simulink model "single_track"  (R2021a)
settings: Solver=VariableStepAuto  StartTime=0.0  StopTime=80  FixedStep=0.001  RelTol=1e-3
libraries: pid_lib x1
settings Model: Creator=ouafo  LastModifiedBy=ouafo

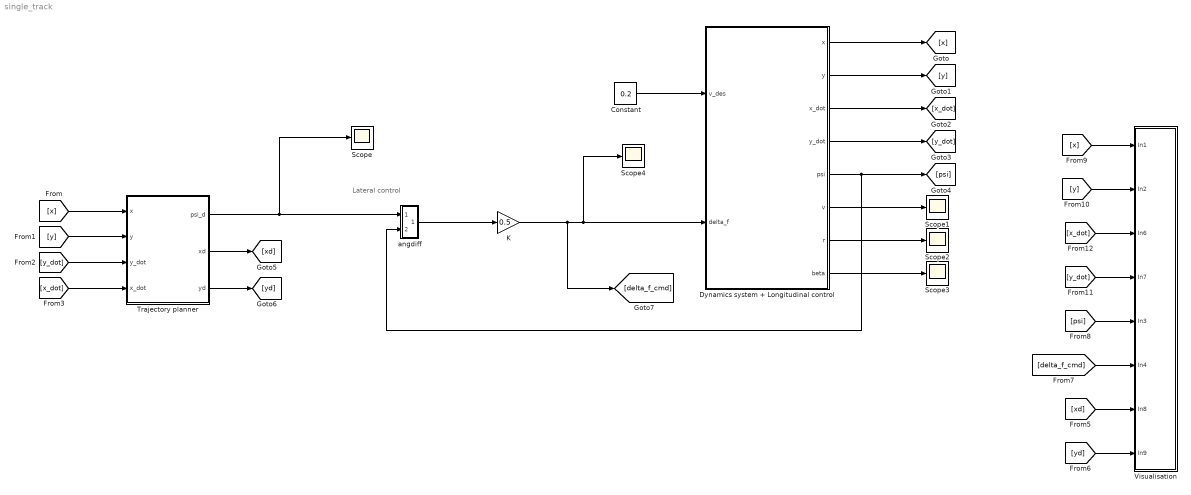
== system single_track ==
  note: Lateral control
  Constant : Constant  Value=0.2
  Dynamics system + Longitudinal control : Subsystem
  K : Gain  Gain=0.5
  Scope{,1..4} (5 alike) : Scope
  Trajectory planner : Subsystem
  Visualisation : Subsystem
  angdiff : Subsystem
  wires:
  Constant/1 -> Dynamics system + Longitudinal control/1(v_des)
  Dynamics system + Longitudinal control/1(x) -> [x]
  Dynamics system + Longitudinal control/2(y) -> [y]
  Dynamics system + Longitudinal control/3(x_dot) -> [x_dot]
  Dynamics system + Longitudinal control/4(y_dot) -> [y_dot]
  Dynamics system + Longitudinal control/5(psi) -> angdiff/2(-), [psi]
  Dynamics system + Longitudinal control/6(v) -> Scope1/1
  Dynamics system + Longitudinal control/7(r) -> Scope2/1
  Dynamics system + Longitudinal control/8(beta) -> Scope3/1
  [x] -> Trajectory planner/1(x)
  [y] -> Trajectory planner/2(y)
  [y_dot] -> Trajectory planner/3(y_dot)
  [x_dot] -> Trajectory planner/4(x_dot)
  Trajectory planner/2(xd) -> [xd]
  Trajectory planner/3(yd) -> [yd]
  angdiff/1(e) -> K/1
  [x] -> Visualisation/1(In1)
  [y] -> Visualisation/2(In2)
  [yd] -> Visualisation/8(In9)
  [xd] -> Visualisation/7(In8)
  [x_dot] -> Visualisation/3(In6)
  [y_dot] -> Visualisation/4(In7)
  [delta_f_cmd] -> Visualisation/6(In4)
  [psi] -> Visualisation/5(In3)
  Trajectory planner/1(psi_d) -> Scope/1, angdiff/1(+)
  K/1 -> [delta_f_cmd], Scope4/1, Dynamics system + Longitudinal control/2(delta_f)

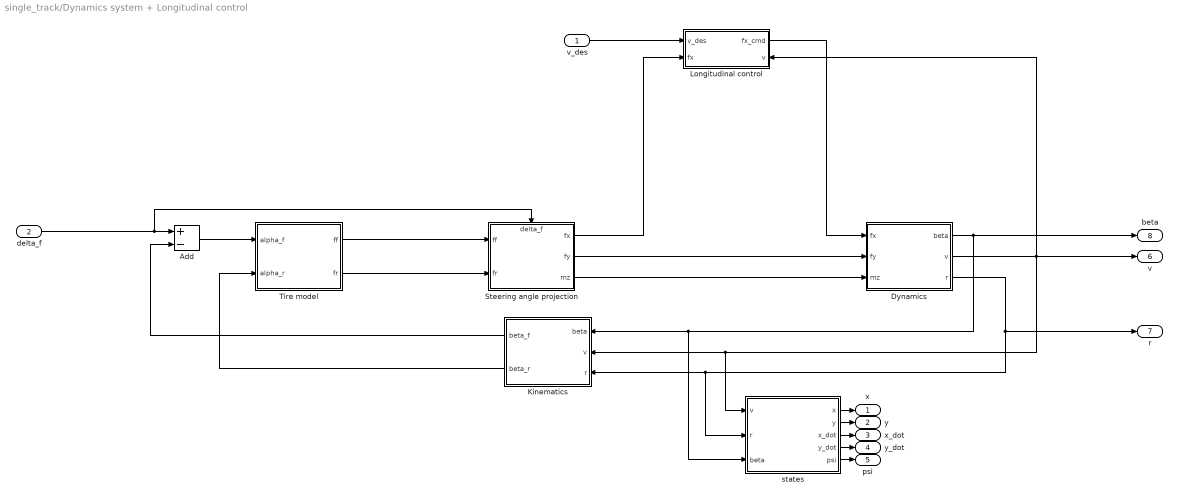
== system single_track/Dynamics system + Longitudinal control ==
  v_des : Inport
  delta_f : Inport  Port=2
  Add : Sum  Inputs=+-
  Dynamics : Subsystem
  Kinematics : Subsystem
  Longitudinal control : Subsystem
      settings: PortSchema="{\"entries\":[{\"content\":{\"sides\":[{\"content\":{\"connectorIds\":[\"In1\",\"In2\"]},\"type\":\"ConnectorPlacement.EquallySpacedRectSide\",\"uuid\":\"998833cc-1ae3-458a-8afb-96cc18db8c80\"},{\"content\":{\"connectorIds\":[\"Out1\",\"In3\"],\"side\":\"RIGHT\"},\"type\":\"ConnectorPlacement.EquallySpacedRectSide\",\"uuid\":\"fcb5fd6e-7c15-4d63-8239-7525f445e8c5\"},{\"content\":{\"connectorIds\":[],\"side\":\"TOP\"},\"type\":\"ConnectorPlacement.EquallySpacedRectSide\",\"uuid\":\"70c6e347-3bc2-4202-b834-379cf179dd08\"},{\"content\":{\"connectorIds\":[],\"side\":\"BOTTOM\"},\"type\":\"ConnectorPlacement.EquallySpacedRectSide\",\"uuid\":\"2cc4168b-3eb3-494f-b0d0-8a728c963cb1\"}]},\"type\":\"ConnectorPlacement.EquallySpacedConnector\",\"uuid\":\"1cd2931d-9394-40f3-bda0-3ecfedd53b05\"}],\"packageUris\":[\"http://schema.mathworks.com/mf0/Connector/R2020b\"],\"version\":\"1.0\"}"
  Steering angle projection : Subsystem
      settings: PortSchema="{\"entries\":[{\"content\":{\"sides\":[{\"content\":{\"connectorIds\":[\"In1\",\"In2\"]},\"type\":\"ConnectorPlacement.EquallySpacedRectSide\",\"uuid\":\"851b8f0b-7850-4432-b3a6-e49d1b849a22\"},{\"content\":{\"connectorIds\":[\"Out1\",\"Out2\",\"Out3\"],\"side\":\"RIGHT\"},\"type\":\"ConnectorPlacement.EquallySpacedRectSide\",\"uuid\":\"60b21c17-1cf9-454c-9b20-5b400b47ede1\"},{\"content\":{\"connectorIds\":[\"In3\"],\"side\":\"TOP\"},\"type\":\"ConnectorPlacement.EquallySpacedRectSide\",\"uuid\":\"9c5c9653-2b7a-48f5-af80-1cee6375c418\"}]},\"type\":\"ConnectorPlacement.EquallySpacedConnector\",\"uuid\":\"bd97c71a-a528-4f5e-9945-06be100bb47e\"}],\"packageUris\":[\"http://schema.mathworks.com/mf0/Connector/R2020b\"],\"version\":\"1.0\"}"
  Tire model : Subsystem
  states : Subsystem
  x : Outport
  y : Outport  Port=2
  x_dot : Outport  Port=3
  y_dot : Outport  Port=4
  psi : Outport  Port=5
  v : Outport  Port=6
  r : Outport  Port=7
  beta : Outport  Port=8
  wires:
  Longitudinal control/1(fx_cmd) -> Dynamics/1(fx)
  Tire model/2(fr) -> Steering angle projection/2(fr)
  Tire model/1(ff) -> Steering angle projection/1(ff)
  states/1(x) -> x/1
  states/3(x_dot) -> x_dot/1
  delta_f/1 -> Steering angle projection/3(delta_f), Add/1
  Dynamics/2(v) -> v/1, states/1(v), Kinematics/2(v), Longitudinal control/3(v)
  Kinematics/1(beta_f) -> Add/2
  Kinematics/2(beta_r) -> Tire model/2(alpha_r)
  v_des/1 -> Longitudinal control/1(v_des)
  states/2(y) -> y/1
  Add/1 -> Tire model/1(alpha_f)
  Steering angle projection/3(mz) -> Dynamics/3(mz)
  states/4(y_dot) -> y_dot/1
  Dynamics/1(beta) -> beta/1, Kinematics/1(beta), states/3(beta)
  Steering angle projection/1(fx) -> Longitudinal control/2(fx)
  Dynamics/3(r) -> r/1, Kinematics/3(r), states/2(r)
  Steering angle projection/2(fy) -> Dynamics/2(fy)
  states/5(psi) -> psi/1

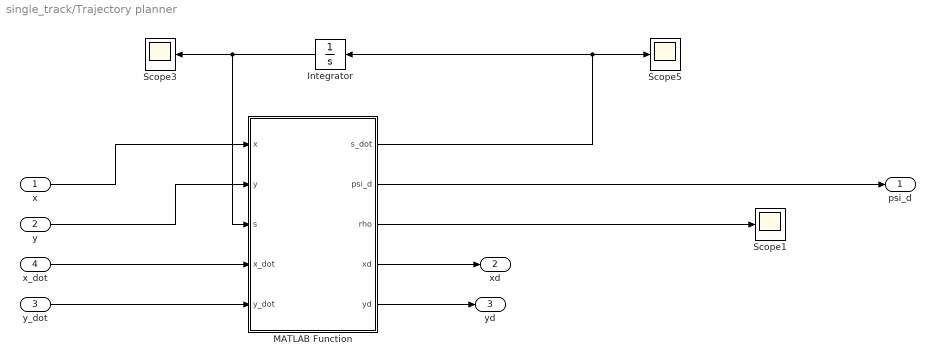
== system single_track/Trajectory planner ==
  x : Inport
  y : Inport  Port=2
  y_dot : Inport  Port=3
  x_dot : Inport  Port=4
  Integrator : Integrator  InitialCondition=-2
  MATLAB Function : MATLAB Function  TreatAsAtomicUnit=on
  Scope1 : Scope
  Scope3 : Scope
  Scope5 : Scope
  psi_d : Outport
  xd : Outport  Port=2
  yd : Outport  Port=3
  wires:
  x/1 -> MATLAB Function/1(x)
  y/1 -> MATLAB Function/2(y)
  y_dot/1 -> MATLAB Function/5(y_dot)
  x_dot/1 -> MATLAB Function/4(x_dot)
  MATLAB Function/1(s_dot) -> Integrator/1, Scope5/1
  Integrator/1 -> MATLAB Function/3(s), Scope3/1
  MATLAB Function/2(psi_d) -> psi_d/1
  MATLAB Function/3(rho) -> Scope1/1
  MATLAB Function/4(xd) -> xd/1
  MATLAB Function/5(yd) -> yd/1

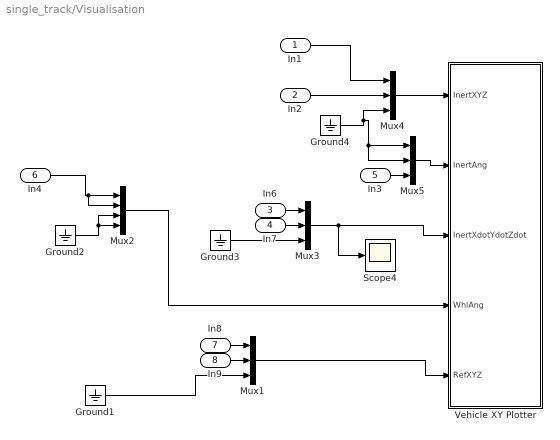
== system single_track/Visualisation ==
  In1 : Inport  PortDimensions=1
  In2 : Inport  Port=2  PortDimensions=1
  In6 : Inport  Port=3  PortDimensions=1
  In7 : Inport  Port=4  PortDimensions=1
  In3 : Inport  Port=5  PortDimensions=1
  In4 : Inport  Port=6  PortDimensions=1
  In8 : Inport  Port=7  PortDimensions=1
  In9 : Inport  Port=8  PortDimensions=1
  Ground{1..4} (4 alike) : Ground
  Mux{1,3..5} (4 alike) : Mux  Inputs=3
  Mux2 : Mux
  Scope4 : Scope
  Vehicle XY Plotter : Subsystem  AncestorBlock=vehdynlibviscommon/Vehicle XY Plot Configuration  mask(Vehicle XY Plotter){extRef=on, extStats=off, extTireF=off, a=0.5, b=0.5, w=1, figBorder=8, bufferSize=1024*100, velNorm=1, tireFNorm=1000, pltDT=0.5}
      mask prompts: extRef "Plot path reference, extRef"; extStats "Display speed, RPM and Gear"; extTireF "Display tire forces"; a "Distance to front axle from CG, a [m]:"; b "Distance to rear axle from CG, b [m]:"; w "Track width, w [m]:"; figBorder "Distance to figure borders, figBorder [m]:"; bufferSize "Path buffer sampe size, bufferSize []:"; velNorm "Velocity vector scaling, velNorm [m*s/m]:"; tireFNorm "Tire force vector scaling, tireFNorm [m/N]:"; pltDT "Plot update rate, pltDT [s]:"
      mask help:
      | This block will display a MATLAB figure which indicates the vehicle path, current position and heading velocity.
      | An optional path reference is also provided.
      mask init:
      | block = gcb;
      | if autoblkschecksimstopped(block)
      |     ParamNames = {'extRef';'extStats';'extTireF';'extTireF'};
      |     PortNames = {'RefXYZ';'Stats';'TireFx';'TireFy'};
      |     for idx=1:length(PortNames)
      |         InportOption  = {'built-in/Ground', [PortNames{idx}, ' Ground'];...
      |             'built-in/Inport',PortNames{idx}};
      |         if ~strcmp(get_param(block,ParamNames{idx}),'on')
      |             NewBlkHdl = autoblksreplaceblock(block, InportOption, 1);
      |             set_param(NewBlkHdl, 'ShowName', 'off');
      |         else
      |             autoblksreplaceblock(block, InportOption, 2);
      |         end
      |     end
      |     InportNames = {'InertXYZ';'InertAng';'InertXdotYdotZdot';'WhlAng';'RefXYZ';'Stats';'TireFx';'TireFy'};
      |     FoundNames = get_param(find_system(block, 'LookUnderMasks', 'all', 'SearchDepth', 1, 'FollowLinks', 'on', 'BlockType', 'Inport'), 'Name');
      |     [~,PortI] = intersect(InportNames, FoundNames);
      |     PortI = sort(PortI);
      |     for idx = 1:length(PortI)
      |         set_param([block, '/', InportNames{PortI(idx)}], 'Port', num2str(idx));
      |     end
      | end
      mask TypeOptions a: Vehicle XY Plotter/a
      mask TypeOptions b: Vehicle XY Plotter/b
      mask TypeOptions w: Vehicle XY Plotter/w
      mask TypeOptions figBorder: Vehicle XY Plotter/figBorder
      mask TypeOptions bufferSize: Vehicle XY Plotter/bufferSize
      mask TypeOptions velNorm: Vehicle XY Plotter/velNorm
      mask TypeOptions tireFNorm: Vehicle XY Plotter/tireFNorm
      mask DialogControl Container3 Prompt: Plot and Display Options
  wires:
  Mux2/1 -> Vehicle XY Plotter/4(WhlAng)
  Ground1/1 -> Mux1/3
  Mux3/1 -> Scope4/1, Vehicle XY Plotter/3(InertXdotYdotZdot)
  Ground3/1 -> Mux3/3
  In7/1 -> Mux3/2
  Mux4/1 -> Vehicle XY Plotter/1(InertXYZ)
  Mux1/1 -> Vehicle XY Plotter/5(RefXYZ)
  In1/1 -> Mux4/1
  In3/1 -> Mux5/3
  In2/1 -> Mux4/2
  In6/1 -> Mux3/1
  In4/1 -> Mux2/2, Mux2/1
  In8/1 -> Mux1/1
  Ground2/1 -> Mux2/3, Mux2/4
  Ground4/1 -> Mux5/2, Mux5/1, Mux4/3
  Mux5/1 -> Vehicle XY Plotter/2(InertAng)
  In9/1 -> Mux1/2

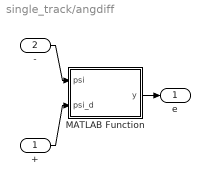
== system single_track/angdiff ==
  + : Inport
  - : Inport  Port=2
  MATLAB Function : MATLAB Function  TreatAsAtomicUnit=on
  e : Outport
  wires:
  +/1 -> MATLAB Function/2(psi_d)
  MATLAB Function/1(y) -> e/1
  -/1 -> MATLAB Function/1(psi)

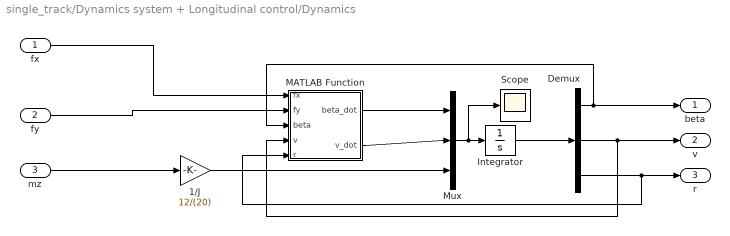
== system single_track/Dynamics system + Longitudinal control/Dynamics ==
  fx : Inport
  fy : Inport  Port=2
  mz : Inport  Port=3
  1/J : Gain  Gain=12/(20)
  Demux : Demux  Outputs=3
  Integrator : Integrator  InitialCondition=[0 0.2 0]
  MATLAB Function : MATLAB Function  TreatAsAtomicUnit=on
  Mux : Mux  Inputs=3
  Scope : Scope
  beta : Outport
  v : Outport  Port=2
  r : Outport  Port=3
  wires:
  Integrator/1 -> Demux/1
  Demux/1 -> beta/1, MATLAB Function/3(beta)
  Demux/2 -> MATLAB Function/4(v), v/1
  Demux/3 -> MATLAB Function/5(r), r/1
  mz/1 -> 1/J/1
  Mux/1 -> Scope/1, Integrator/1
  1/J/1 -> Mux/3
  MATLAB Function/2(v_dot) -> Mux/2
  MATLAB Function/1(beta_dot) -> Mux/1
  fx/1 -> MATLAB Function/1(fx)
  fy/1 -> MATLAB Function/2(fy)

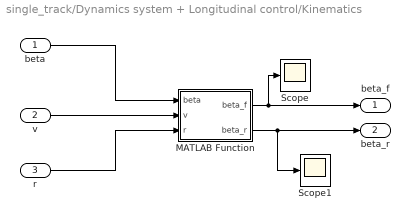
== system single_track/Dynamics system + Longitudinal control/Kinematics ==
  beta : Inport
  v : Inport  Port=2
  r : Inport  Port=3
  MATLAB Function : MATLAB Function  TreatAsAtomicUnit=on
  Scope : Scope
  Scope1 : Scope
  beta_f : Outport
  beta_r : Outport  Port=2
  wires:
  beta/1 -> MATLAB Function/1(beta)
  v/1 -> MATLAB Function/2(v)
  r/1 -> MATLAB Function/3(r)
  MATLAB Function/2(beta_r) -> Scope1/1, beta_r/1
  MATLAB Function/1(beta_f) -> Scope/1, beta_f/1

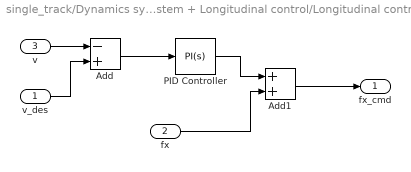
== system single_track/Dynamics system + Longitudinal control/Longitudinal control ==
  v_des : Inport
  fx : Inport  Port=2
  v : Inport  Port=3
  Add : Sum  Inputs=-+
  Add1 : Sum
  PID Controller : pid_lib/PID Controller  Controller=PI  Form=Parallel  TimeDomain=Continuous-time  UseExternalTs=off  SampleTime=-1  IntegratorMethod=Forward Euler  FilterMethod=Forward Euler  ControllerParametersSource=internal  P=40.8208009338721  I=35.2403929925848  D=0  UseFilter=on  N=100  TunerSelectOption=Transfer Function Based (PID Tuner App)  InitialConditionSource=internal  InitialConditionForIntegrator=0  InitialConditionForFilter=0  DifferentiatorICPrevScaledInput=0  ExternalReset=none  TrackingMode=off  Kt=1  LimitOutput=off  SatLimitsSource=internal  UpperSaturationLimit=inf  LowerSaturationLimit=-inf  LinearizeAsGain=on  AntiWindupMode=none  Kb=1  POutMin=[]  POutMax=[]  IOutMin=[]  IOutMax=[]  DOutMin=[]  DOutMax=[]  NOutMin=[]  NOutMax=[]  SumOutMin=[]  SumOutMax=[]  SaturationOutMin=[]  SaturationOutMax=[]  PParamMin=[]  PParamMax=[]  IParamMin=[]  IParamMax=[]  DParamMin=[]  DParamMax=[]  NParamMin=[]  NParamMax=[]  KbParamMin=[]  KbParamMax=[]  KtParamMin=[]  KtParamMax=[]  KbOutMin=[]  KbOutMax=[]  KtOutMin=[]  KtOutMax=[]  IntegratorOutMin=[]  IntegratorOutMax=[]  FilterOutMin=[]  FilterOutMax=[]  SumI1OutMin=[]  SumI1OutMax=[]  SumI2OutMin=[]  SumI2OutMax=[]  SumI3OutMin=[]  SumI3OutMax=[]  SumI4OutMin=[]  SumI4OutMax=[]  SumDOutMin=[]  SumDOutMax=[]  DifferentiatorOutMin=[]  DifferentiatorOutMax=[]  FilterDiffOutCoefMin=[]  FilterDiffOutCoefMax=[]  ReciprocalOutMin=[]  ReciprocalOutMax=[]  SumDenOutMin=[]  SumDenOutMax=[]  SumNumOutMin=[]  SumNumOutMax=[]  DivideOutMin=[]  DivideOutMax=[]  UdiffTsProdOutMin=[]  UdiffTsProdOutMax=[]  NTsProdOutMin=[]  NTsProdOutMax=[]  UintegralTsProdOutMin=[]  UintegralTsProdOutMax=[]  UngainTsProdOutMin=[]  UngainTsProdOutMax=[]  IntegratorContinuousStateAttributes=''  IntegratorStateMustResolveToSignalObject=off  IntegratorRTWStateStorageClass=Auto  FilterContinuousStateAttributes=''  FilterStateMustResolveToSignalObject=off  FilterRTWStateStorageClass=Auto  ParallelPVariant=InternalParameters  IdealPVariant=Disabled  IVariant=InternalParameters  DVariant=Disabled  IntegratorVariant=Continuous  SatVariant=Disabled  AWVariant=Passthrough  PCopyVariant=Disabled  TRVariant=Disabled  FdbkBlocksVariant=Forward  IdealPFdbkVariant=Disabled  SatFdbkVariant=Disabled  DerivativeFilterVariant=Disabled  NVariant=Disabled  NCopyVariant=Disabled_SignalSpec  FilterICVariant=Disabled  IntegratorICVariant=InternalICs  ExternalResetVariant=Disabled  TRSumVariant=Passthrough  SumFdbkVariant=Disabled  SumVariant=Sum_PI  TsampFilterVariant=InternalTs  TsampNgainVariant=Passthrough  TsampIntegralVariant=Passthrough  ExternalSaturationOutDataTypeStr=Inherit: Same as second input
  fx_cmd : Outport
  wires:
  v/1 -> Add/1
  v_des/1 -> Add/2
  Add/1 -> PID Controller/1
  PID Controller/1 -> Add1/1
  fx/1 -> Add1/2
  Add1/1 -> fx_cmd/1

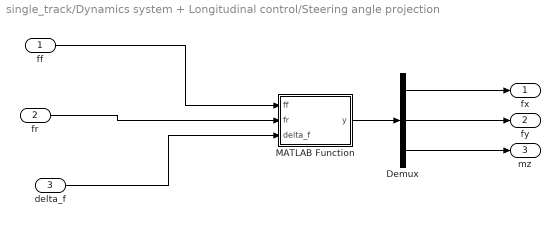
== system single_track/Dynamics system + Longitudinal control/Steering angle projection ==
  ff : Inport
  fr : Inport  Port=2
  delta_f : Inport  Port=3
  Demux : Demux  Outputs=3
  MATLAB Function : MATLAB Function  TreatAsAtomicUnit=on
  fx : Outport
  fy : Outport  Port=2
  mz : Outport  Port=3
  wires:
  ff/1 -> MATLAB Function/1(ff)
  fr/1 -> MATLAB Function/2(fr)
  delta_f/1 -> MATLAB Function/3(delta_f)
  MATLAB Function/1(y) -> Demux/1
  Demux/1 -> fx/1
  Demux/2 -> fy/1
  Demux/3 -> mz/1

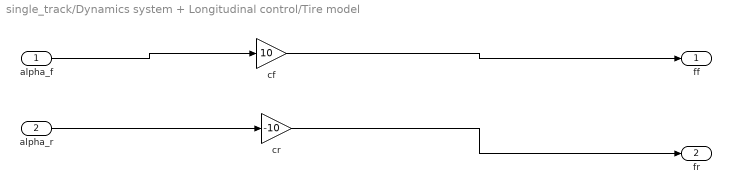
== system single_track/Dynamics system + Longitudinal control/Tire model ==
  alpha_f : Inport
  alpha_r : Inport  Port=2
  cf : Gain  Gain=10
  cr : Gain  Gain=-10
  ff : Outport
  fr : Outport  Port=2
  wires:
  alpha_f/1 -> cf/1
  cf/1 -> ff/1
  alpha_r/1 -> cr/1
  cr/1 -> fr/1

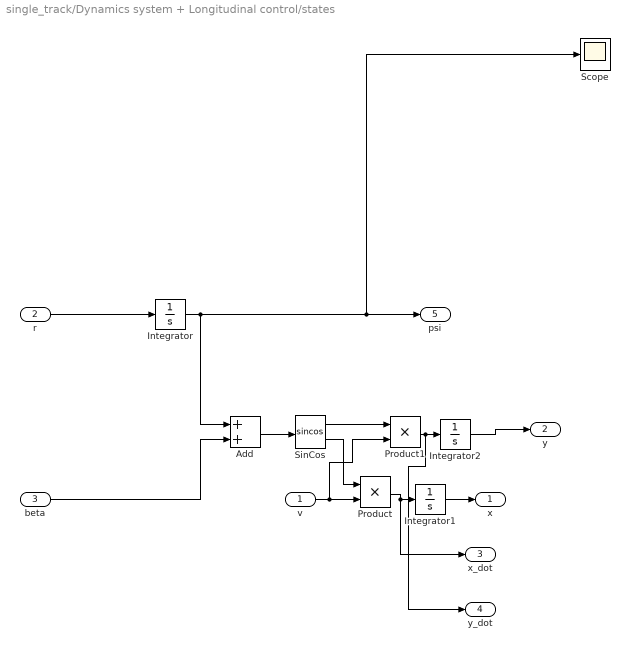
== system single_track/Dynamics system + Longitudinal control/states ==
  v : Inport
  r : Inport  Port=2
  beta : Inport  Port=3
  Add : Sum
  Integrator : Integrator  UpperSaturationLimit=2*pi  LowerSaturationLimit=0
  Integrator1 : Integrator  InitialCondition=-6
  Integrator2 : Integrator  InitialCondition=-5
  Product : Product
  Product1 : Product
  Scope : Scope
  SinCos : Trigonometry  Operator=sincos
  x : Outport
  y : Outport  Port=2
  x_dot : Outport  Port=3
  y_dot : Outport  Port=4
  psi : Outport  Port=5
  wires:
  r/1 -> Integrator/1
  beta/1 -> Add/2
  Add/1 -> SinCos/1
  v/1 -> Product1/2, Product/2
  SinCos/2 -> Product/1
  Integrator1/1 -> x/1
  Product/1 -> x_dot/1, Integrator1/1
  SinCos/1 -> Product1/1
  Product1/1 -> y_dot/1, Integrator2/1
  Integrator2/1 -> y/1
  Integrator/1 -> Scope/1, psi/1, Add/1

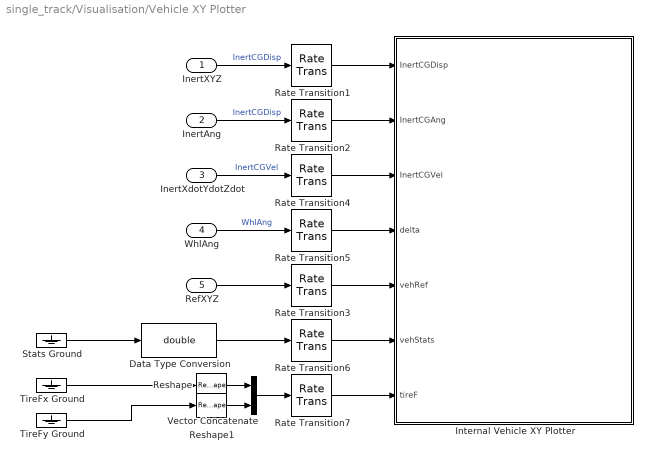
== system single_track/Visualisation/Vehicle XY Plotter ==
  InertXYZ : Inport
  InertAng : Inport  Port=2
  InertXdotYdotZdot : Inport  Port=3
  WhlAng : Inport  Port=4
  RefXYZ : Inport  Port=5
  Data Type Conversion : DataTypeConversion  OutDataTypeStr=double
  Internal Vehicle XY Plotter : MATLAB Function  InitFcn=|  StopFcn=|  TreatAsAtomicUnit=on  mask(Vehicle XY Plotter){bufferSize=bufferSize, w=w, a=a, b=b, figBorder=figBorder, velNorm=velNorm, tireFNorm=tireFNorm}
      InitFcn=|
      | if ~isempty(findobj(allchild(groot), 'flat', 'type', 'figure', 'Name', 'Vehicle Position'))
      |   close gcf;
      | end
      StopFcn=|
      | if ~isempty(findobj(allchild(groot), 'flat', 'type', 'figure', 'Name', 'Vehicle Position'))
      | axis auto;
      | axis equal;
      | end
      mask prompts: bufferSize "Path buffer sampe size, bufferSize []:"; w "Track width, w [m]:"; a "Distance to front axle from CG, a [m]:"; b "Distance to rear axle from CG, b [m]:"; figBorder "Distance to figure borders during run time, figBorder [m]:"; velNorm "Velocity vector scaling, velNorm [m*s/m]:"; tireFNorm "Tire force vector scaling, tireFNorm [m/N]:"
      mask help: This block will display a MATLAB figure which indicates the vehicle path, current position and heading velocity.
      mask init:
      | [~] = vehdynicon('vehdyn2Dplot',gcb,0)
      | scrnSize = get(groot,'Screensize');
      | figWidth = floor(scrnSize(3)./3);
  Rate Transition{1..7} (7 alike) : RateTransition  Deterministic=off  OutPortSampleTime=pltDT
  Reshape : Reshape  OutputDimensionality=Row vector (2-D)
  Reshape1 : Reshape  OutputDimensionality=Row vector (2-D)
  Stats Ground : Ground
  TireFx Ground : Ground
  TireFy Ground : Ground
  Vector Concatenate : Concatenate  Mode=Multidimensional array
  wires:
  Rate Transition2/1 -> Internal Vehicle XY Plotter/2(InertCGAng)
  Vector Concatenate/1 -> Rate Transition7/1
  Reshape1/1 -> Vector Concatenate/2
  Reshape/1 -> Vector Concatenate/1
  RefXYZ/1 -> Rate Transition3/1
  Rate Transition7/1 -> Internal Vehicle XY Plotter/7(tireF)
  Data Type Conversion/1 -> Rate Transition6/1
  Rate Transition6/1 -> Internal Vehicle XY Plotter/6(vehStats)
  Rate Transition5/1 -> Internal Vehicle XY Plotter/4(delta)
  Rate Transition4/1 -> Internal Vehicle XY Plotter/3(InertCGVel)
  Rate Transition1/1 -> Internal Vehicle XY Plotter/1(InertCGDisp)
  Rate Transition3/1 -> Internal Vehicle XY Plotter/5(vehRef)
  WhlAng/1 -> Rate Transition5/1  "WhlAng"
  InertXYZ/1 -> Rate Transition1/1  "InertCGDisp"
  InertXdotYdotZdot/1 -> Rate Transition4/1  "InertCGVel"
  InertAng/1 -> Rate Transition2/1  "InertCGDisp"
  TireFx Ground/1 -> Reshape/1
  TireFy Ground/1 -> Reshape1/1
  Stats Ground/1 -> Data Type Conversion/1

== matlab function single_track/Dynamics system + Longitudinal control/Kinematics/MATLAB Function ==
  data: beta input; beta_f output; v input; r input; beta_r output
function [beta_f, beta_r] = fcn(beta,v,r)

lf = 0.5;
lr = 0.5;



beta_f = atan( tan(beta) + (lf*r)/(v*cos(beta)));
beta_r = atan( tan(beta) - (lr*r)/(v*cos(beta)));

== matlab function single_track/Dynamics system + Longitudinal control/Dynamics/MATLAB Function ==
  data: fx input; beta_dot output; fy input; beta input; v input; v_dot output; r input
function [beta_dot, v_dot] = fcn(fx, fy, beta, v, r)

m = 10; % mass of the car

beta_dot = -(fx*sin(beta) - fy*cos(beta) + m*r*v) / (m * v);
v_dot = (fx * cos(beta) + fy * sin(beta)) / m;

== matlab function single_track/Dynamics system + Longitudinal control/Steering angle projection/MATLAB Function ==
  data: ff input; y output; fr input; delta_f input
function y = fcn(ff, fr, delta_f)

lf = 0.5;
lr = 0.5;

A = [-sin(delta_f) 0;cos(delta_f) 1;lf*cos(delta_f) -lr];

y = A * [ff;fr];

== matlab function single_track/angdiff/MATLAB Function ==
  data: psi input; y output; psi_d input
function y = fcn(psi,psi_d)

y = angdiff(psi,psi_d);

== matlab function single_track/Trajectory planner/MATLAB Function ==
  settings: updateMethod=DISCRETE
  data: x input; y input; s input; s_dot output; x_dot input; y_dot input; psi_d output; rho output; xd output; yd output
function [s_dot,psi_d,rho,xd,yd] = fcn(x, y,s, x_dot, y_dot)

% coder.extrinsic('getframe');
% coder.extrinsic('frame2im');
% coder.extrinsic('rgb2ind');
% coder.extrinsic('imwrite');
% persistent index;

d = 1; % look-ahead distance
gamma = 1;



% xd = 10 + sin(s*0.01);
% yd = -20 + 10*sin(s*0.01/2);


xd = s;
yd = s^3;



%xd = 20 + 10*sin(s/10);
%yd = 0 - 10*cos(s/10);

dx= x-xd;
dy= y-yd;



rho = sqrt(dx*dx+dy*dy);


%s_dot = (dx*x_dot+dy*y_dot+gamma*rho*(rho-d))/(dx*cos(s/10)+dy*sin(s/10));
s_dot = (dx*x_dot+dy*y_dot+gamma*rho*(rho-d))/(dx + 3 *dy*s^2);

psi_d = atan2(-dy,-dx);

== matlab function single_track/Visualisation/Vehicle XY Plotter/Internal Vehicle XY Plotter ==
  data: InertCGDisp input; InertCGAng input double; InertCGVel input; delta input size=4; vehRef input size=3; vehStats input size=[2,1]; tireF input size=[2,4]; bufferSize parameter; figBorder parameter; figWidth parameter; w parameter; a parameter; b parameter; extRef parameter; extStats parameter; extTireF parameter; velNorm parameter size=1 [eps..]; tireFNorm parameter size=1 [eps..]
function vdynplot(InertCGDisp,InertCGAng,InertCGVel,delta,vehRef,vehStats,tireF,bufferSize,figBorder, figWidth, w, a, b,extRef, extStats, extTireF,velNorm, tireFNorm)
coder.allowpcode('plain')
% Copyright 2017-2020 The MathWorks, Inc.
coder.extrinsic('vdynXYplot');
coder.extrinsic('getframe');
coder.extrinsic('frame2im');
coder.extrinsic('rgb2ind');
coder.extrinsic('imwrite');
persistent index;
vdynXYplot(InertCGDisp,InertCGAng,InertCGVel,delta,vehRef,vehStats,tireF,bufferSize,figBorder, figWidth, w, a, b,extRef, extStats, extTireF,velNorm,tireFNorm)

filename = 'test.gif';

frame = getframe(gcf);
im = frame2im(frame);
[imind,cm] = rgb2ind(im,256);
if isempty(index)
    imwrite(imind,cm,filename,'gif','Loopcount',inf,'DelayTime', .1);
    index = 0;
else
    imwrite(imind,cm,filename,'gif','WriteMode','append','DelayTime', .1);
    index = index+1;
end
end
